simulink model "segway_project"  (R2015a)
settings: Solver=ode3  StartTime=0.0  StopTime=inf  FixedStep=Ts  RelTol=1e-3
values from neighbouring files (symbols this model uses):
  K = lqr(A,B,Q,R)    [Segway_Setup.m]
  Rw = 0.0216    [Segway_Setup.m]
  Ts = 0.005    [Segway_Setup.m]
libraries: MinSegLibrary_M1V4 x2, simulink x1, RASPlib x1
settings Model: ExtModeTrigDuration=2  Creator=Johnsg7  LastModifiedBy=Johnsg7
settings OptimizationCC: OptimizeModelRefInitCode=on  LifeSpan=1
settings DebuggingCC: UnderspecifiedInitializationDetection=Classic  MergeDetectMultiDrivingBlocksExec=none
settings HardwareCC: ProdBitPerInt=16  ProdBitPerPointer=8  ProdIntDivRoundTo=Zero  ProdEndianess=LittleEndian  ProdWordSize=8  ProdHWDeviceType=Atmel->AVR
settings RTWCC: SystemTargetFile=realtime.tlc  GenerateMakefile=off  TemplateMakefile=realtime.tmf  Description=Run on Target Hardware  RTWVerbose=off
settings ERTTargetCC: CombineOutputUpdateFcns=off  ExtModeTransport=3  ExtModeMexFile=ext_serial_win32_comm_rtt  ExtModeMexArgs=0 1 9600  ERTSrcFileBannerTemplate=realtime_code_template.cgt  ERTHdrFileBannerTemplate=realtime_code_template.cgt  ERTDataSrcFileTemplate=realtime_code_template.cgt  ERTDataHdrFileTemplate=realtime_code_template.cgt  ERTCustomFileTemplate=realtime_file_process.tlc

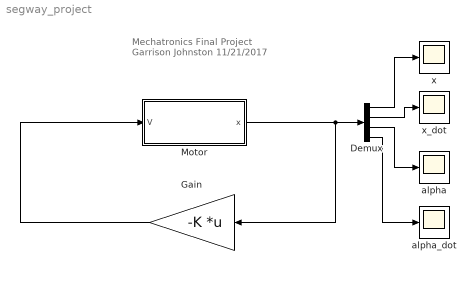
== system segway_project ==
  note: Mechatronics Final Project
      | Garrison Johnston
      | 11/21/2017
  Demux : Demux
  Gain : Gain  Gain=-K  Multiplication=Matrix(K*u)
  Motor : Subsystem
  alpha : Scope
      settings: SaveName=ScopeData3
  alpha_dot : Scope
      settings: SaveName=ScopeData4
  x : Scope
  x_dot : Scope
      settings: SaveName=ScopeData2
  wires:
  Gain/1 -> Motor/1(V)
  Demux/1 -> x/1
  Demux/2 -> x_dot/1
  Demux/3 -> alpha/1
  Demux/4 -> alpha_dot/1
  Motor/1(x) -> Gain/1, Demux/1

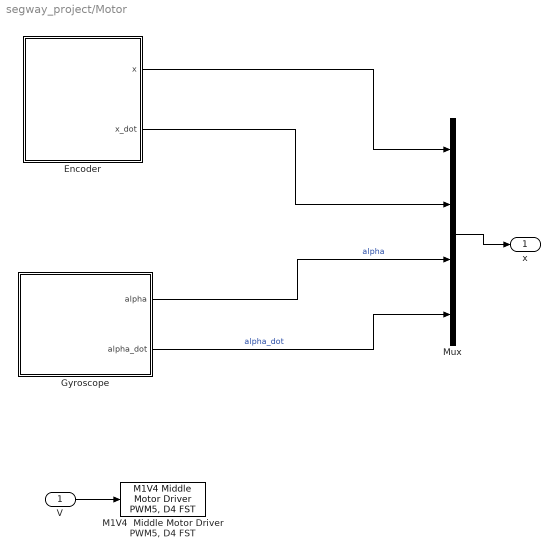
== system segway_project/Motor ==
  V : Inport
  Encoder : Subsystem
  Gyroscope : Subsystem
  "M1V4  Middle Motor Driver PWM5, D4 FST" : MinSegLibrary_M1V4/M1V4  Middle Motor Driver PWM5, D4 FST  Vsupply=7.8
  Mux : Mux
  x : Outport
  wires:
  V/1 -> "M1V4  Middle Motor Driver PWM5, D4 FST"/1
  Mux/1 -> x/1
  Gyroscope/1(alpha) -> Mux/3  "alpha"
  Gyroscope/2(alpha_dot) -> Mux/4  "alpha_dot"
  Encoder/1(x) -> Mux/1
  Encoder/2(x_dot) -> Mux/2

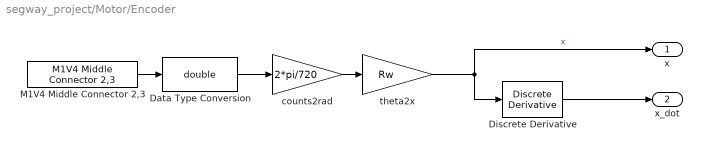
== system segway_project/Motor/Encoder ==
  Data Type Conversion : DataTypeConversion  OutDataTypeStr=double
  Discrete Derivative : simulink/Discrete/Discrete Derivative  gainval=1.0  ICPrevScaledInput=0.0  InputProcessing=Inherited  OutMin=[]  OutMax=[]  OutDataTypeStr=Inherit: Inherit via back propagation  OutDataType=sfix64_En37  OutScaling=[]  DoSatur=off
  M1V4 Middle Connector 2,3 : MinSegLibrary_M1V4/M1V4 Middle Connector 2,3  Encoder=0  PinA=2  PinB=3  PWMFSelect=3  PWMTimer=-1
  counts2rad : Gain  Gain=2*pi/720  ParamDataTypeStr=single
  theta2x : Gain  Gain=Rw  ParamDataTypeStr=single
  x : Outport
  x_dot : Outport  Port=2
  wires:
  theta2x/1 -> x/1, Discrete Derivative/1  "x"
  counts2rad/1 -> theta2x/1
  Discrete Derivative/1 -> x_dot/1
  M1V4 Middle Connector 2,3/1 -> Data Type Conversion/1
  Data Type Conversion/1 -> counts2rad/1

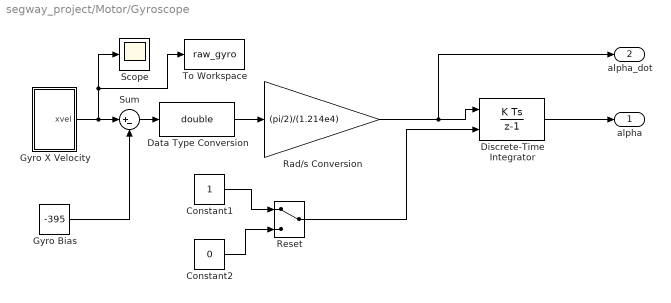
== system segway_project/Motor/Gyroscope ==
  Constant1 : Constant
  Constant2 : Constant  Value=0
  Data Type Conversion : DataTypeConversion  OutDataTypeStr=double
  Discrete-Time Integrator : DiscreteIntegrator  ExternalReset=either  SampleTime=Ts
  Gyro Bias : Constant  Value=-395
  Gyro X Velocity : Subsystem
  Rad/s Conversion : Gain  Gain=(pi/2)/(1.214e4)
  Reset : ManualSwitch
  Scope : Scope
      settings: YMin=-510  YMax=-300
  Sum : Sum  Inputs=|+-
  To Workspace : ToWorkspace  VariableName=raw_gyro  SampleTime=Ts
      settings: Save2DSignal=2-D array (concatenate along first dimension)
  alpha : Outport
  alpha_dot : Outport  Port=2
  wires:
  Discrete-Time Integrator/1 -> alpha/1
  Gyro X Velocity/1(xvel) -> To Workspace/1, Scope/1, Sum/1
  Gyro Bias/1 -> Sum/2
  Rad/s Conversion/1 -> Discrete-Time Integrator/1, alpha_dot/1
  Data Type Conversion/1 -> Rad/s Conversion/1
  Reset/1 -> Discrete-Time Integrator/2
  Constant1/1 -> Reset/1
  Constant2/1 -> Reset/2
  Sum/1 -> Data Type Conversion/1

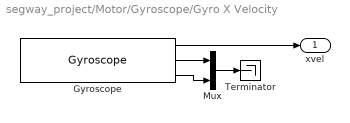
== system segway_project/Motor/Gyroscope/Gyro X Velocity ==
  Gyroscope : RASPlib/Gyroscope  DLPFmode=0
  Mux : Mux  Inputs=2
  Terminator : Terminator
  xvel : Outport
  wires:
  Gyroscope/1 -> xvel/1
  Gyroscope/3 -> Mux/2
  Mux/1 -> Terminator/1
  Gyroscope/2 -> Mux/1
